simulink library "cdsSusSw2"  (Simulink 6.2)
settings Model: LastModifiedBy=rolf

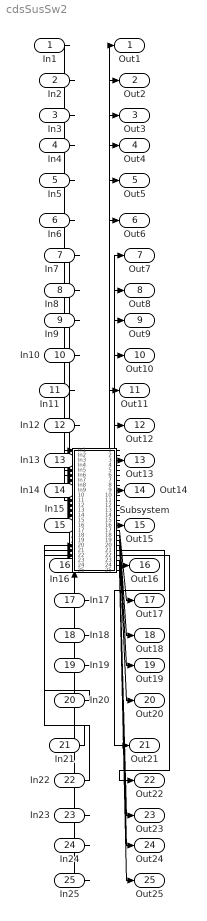
== system cdsSusSw2 ==
  In1 : Inport  Port=1  LatchInput=off
  In2 : Inport  Port=2  LatchInput=off
  In3 : Inport  Port=3  LatchInput=off
  In4 : Inport  Port=4  LatchInput=off
  In5 : Inport  Port=5  LatchInput=off
  In6 : Inport  Port=6  LatchInput=off
  In7 : Inport  Port=7  LatchInput=off
  In8 : Inport  Port=8  LatchInput=off
  In9 : Inport  Port=9  LatchInput=off
  In10 : Inport  Port=10  LatchInput=off
  In11 : Inport  Port=11  LatchInput=off
  In12 : Inport  Port=12  LatchInput=off
  In13 : Inport  Port=13  LatchInput=off
  In14 : Inport  Port=14  LatchInput=off
  In15 : Inport  Port=15  LatchInput=off
  In16 : Inport  Port=16  LatchInput=off
  In17 : Inport  Port=17  LatchInput=off
  In18 : Inport  Port=18  LatchInput=off
  In19 : Inport  Port=19  LatchInput=off
  In20 : Inport  Port=20  LatchInput=off
  In21 : Inport  Port=21  LatchInput=off
  In22 : Inport  Port=22  LatchInput=off
  In23 : Inport  Port=23  LatchInput=off
  In24 : Inport  Port=24  LatchInput=off
  In25 : Inport  Port=25  LatchInput=off
  Subsystem : Subsystem
  Out1 : Outport
  Out2 : Outport  Port=2
  Out3 : Outport  Port=3
  Out4 : Outport  Port=4
  Out5 : Outport  Port=5
  Out6 : Outport  Port=6
  Out7 : Outport  Port=7
  Out8 : Outport  Port=8
  Out9 : Outport  Port=9
  Out10 : Outport  Port=10
  Out11 : Outport  Port=11
  Out12 : Outport  Port=12
  Out13 : Outport  Port=13
  Out14 : Outport  Port=14
  Out15 : Outport  Port=15
  Out16 : Outport  Port=16
  Out17 : Outport  Port=17
  Out18 : Outport  Port=18
  Out19 : Outport  Port=19
  Out20 : Outport  Port=20
  Out21 : Outport  Port=21
  Out22 : Outport  Port=22
  Out23 : Outport  Port=23
  Out24 : Outport  Port=24
  Out25 : Outport  Port=25
  wires:
  Subsystem/1(Out1) -> Out1/1
  In1/1 -> Subsystem/1(In1)
  Subsystem/2(Out2) -> Out2/1
  In2/1 -> Subsystem/2(In2)
  Subsystem/3(Out3) -> Out3/1
  In3/1 -> Subsystem/3(In3)
  Subsystem/4(Out4) -> Out4/1
  In4/1 -> Subsystem/4(In4)
  Subsystem/5(Out5) -> Out5/1
  In5/1 -> Subsystem/5(In5)
  Subsystem/6(Out6) -> Out6/1
  In6/1 -> Subsystem/6(In6)
  Subsystem/7(Out7) -> Out7/1
  In7/1 -> Subsystem/7(In7)
  Subsystem/8(Out8) -> Out8/1
  In8/1 -> Subsystem/8(In8)
  Subsystem/9(Out9) -> Out9/1
  In9/1 -> Subsystem/9(In9)
  Subsystem/10(Out10) -> Out10/1
  In10/1 -> Subsystem/10(In10)
  Subsystem/11(Out11) -> Out11/1
  In11/1 -> Subsystem/11(In11)
  Subsystem/12(Out12) -> Out12/1
  In12/1 -> Subsystem/12(In12)
  Subsystem/13(Out13) -> Out13/1
  In13/1 -> Subsystem/13(In13)
  Subsystem/14(Out14) -> Out14/1
  In14/1 -> Subsystem/14(In14)
  Subsystem/15(Out15) -> Out15/1
  In15/1 -> Subsystem/15(In15)
  Subsystem/16(Out16) -> Out16/1
  In16/1 -> Subsystem/16(In16)
  Subsystem/17(Out17) -> Out17/1
  In17/1 -> Subsystem/17(In17)
  Subsystem/18(Out18) -> Out18/1
  In18/1 -> Subsystem/18(In18)
  Subsystem/19(Out19) -> Out19/1
  In19/1 -> Subsystem/19(In19)
  Subsystem/20(Out20) -> Out20/1
  In20/1 -> Subsystem/20(In20)
  Subsystem/21(Out21) -> Out21/1
  In21/1 -> Subsystem/21(In21)
  Subsystem/22(Out22) -> Out22/1
  In22/1 -> Subsystem/22(In22)
  Subsystem/23(Out23) -> Out23/1
  In23/1 -> Subsystem/23(In23)
  Subsystem/24(Out24) -> Out24/1
  In24/1 -> Subsystem/24(In24)
  Subsystem/25(Out25) -> Out25/1
  In25/1 -> Subsystem/25(In25)

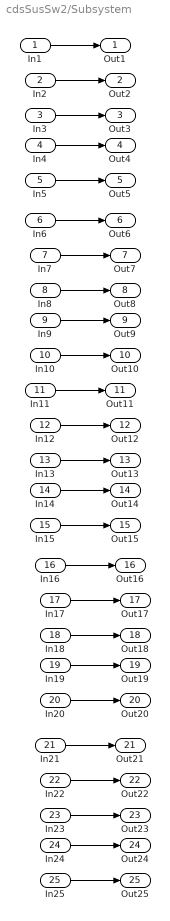
== system cdsSusSw2/Subsystem ==
  In1 : Inport  Port=1  LatchInput=off
  In2 : Inport  Port=2  LatchInput=off
  In3 : Inport  Port=3  LatchInput=off
  In4 : Inport  Port=4  LatchInput=off
  In5 : Inport  Port=5  LatchInput=off
  In6 : Inport  Port=6  LatchInput=off
  In7 : Inport  Port=7  LatchInput=off
  In8 : Inport  Port=8  LatchInput=off
  In9 : Inport  Port=9  LatchInput=off
  In10 : Inport  Port=10  LatchInput=off
  In11 : Inport  Port=11  LatchInput=off
  In12 : Inport  Port=12  LatchInput=off
  In13 : Inport  Port=13  LatchInput=off
  In14 : Inport  Port=14  LatchInput=off
  In15 : Inport  Port=15  LatchInput=off
  In16 : Inport  Port=16  LatchInput=off
  In17 : Inport  Port=17  LatchInput=off
  In18 : Inport  Port=18  LatchInput=off
  In19 : Inport  Port=19  LatchInput=off
  In20 : Inport  Port=20  LatchInput=off
  In21 : Inport  Port=21  LatchInput=off
  In22 : Inport  Port=22  LatchInput=off
  In23 : Inport  Port=23  LatchInput=off
  In24 : Inport  Port=24  LatchInput=off
  In25 : Inport  Port=25  LatchInput=off
  Out1 : Outport
  Out2 : Outport  Port=2
  Out3 : Outport  Port=3
  Out4 : Outport  Port=4
  Out5 : Outport  Port=5
  Out6 : Outport  Port=6
  Out7 : Outport  Port=7
  Out8 : Outport  Port=8
  Out9 : Outport  Port=9
  Out10 : Outport  Port=10
  Out11 : Outport  Port=11
  Out12 : Outport  Port=12
  Out13 : Outport  Port=13
  Out14 : Outport  Port=14
  Out15 : Outport  Port=15
  Out16 : Outport  Port=16
  Out17 : Outport  Port=17
  Out18 : Outport  Port=18
  Out19 : Outport  Port=19
  Out20 : Outport  Port=20
  Out21 : Outport  Port=21
  Out22 : Outport  Port=22
  Out23 : Outport  Port=23
  Out24 : Outport  Port=24
  Out25 : Outport  Port=25
  wires:
  In1/1 -> Out1/1
  In2/1 -> Out2/1
  In3/1 -> Out3/1
  In4/1 -> Out4/1
  In5/1 -> Out5/1
  In6/1 -> Out6/1
  In7/1 -> Out7/1
  In8/1 -> Out8/1
  In9/1 -> Out9/1
  In10/1 -> Out10/1
  In11/1 -> Out11/1
  In12/1 -> Out12/1
  In13/1 -> Out13/1
  In14/1 -> Out14/1
  In15/1 -> Out15/1
  In16/1 -> Out16/1
  In17/1 -> Out17/1
  In18/1 -> Out18/1
  In19/1 -> Out19/1
  In20/1 -> Out20/1
  In21/1 -> Out21/1
  In22/1 -> Out22/1
  In23/1 -> Out23/1
  In24/1 -> Out24/1
  In25/1 -> Out25/1
